simulink subsystem "momentMappingPitchYaw"  (R2026a)
settings: Solver=VariableStepAuto
settings Model: Creator=maxhu  LastModifiedBy=maxhu

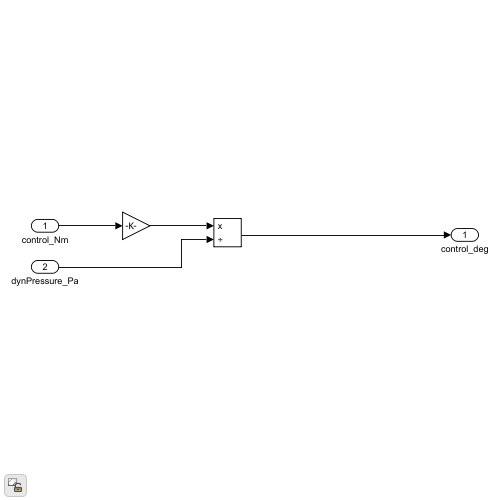
[thumbnail: Simulink's stored preview of the top-level diagram]
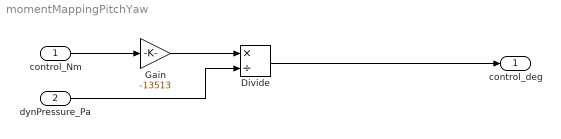
== system momentMappingPitchYaw ==
  control_Nm : Inport
  dynPressure_Pa : Inport  Port=2
  Divide : Product  Inputs=*/
  Gain : Gain  Gain=-13513
  control_deg : Outport
  wires:
  control_Nm/1 -> Gain/1
  dynPressure_Pa/1 -> Divide/2
  Gain/1 -> Divide/1
  Divide/1 -> control_deg/1
